simulink model "Linear_model"  (R2023a)
settings: Solver=VariableStepAuto  StartTime=0.0  StopTime=10.0  RelTol=1e-3
undefined symbols (not defined in the file): A, B, C, K
settings Model: Creator=jonat  LastModifiedBy=jonat

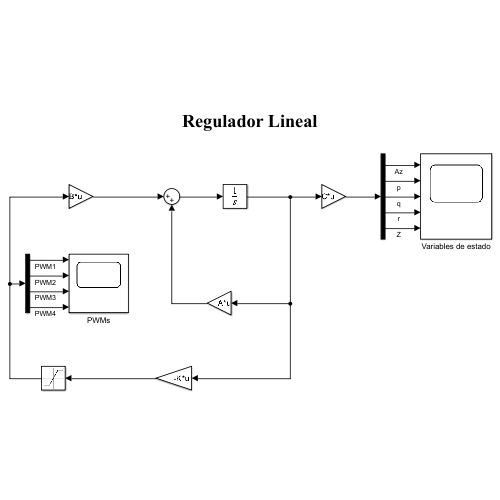
[thumbnail: Simulink's stored preview of the top-level diagram]
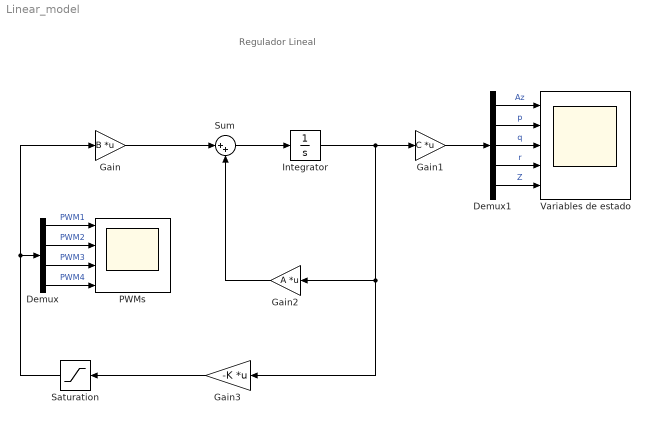
== system Linear_model ==
  note: Regulador Lineal
  Demux : Demux
  Demux1 : Demux  Outputs=5
  Gain : Gain  Gain=B  Multiplication=Matrix(K*u)
  Gain1 : Gain  Gain=C  Multiplication=Matrix(K*u)
  Gain2 : Gain  Gain=A  Multiplication=Matrix(K*u)
  Gain3 : Gain  Gain=-K  Multiplication=Matrix(K*u)
  Integrator : Integrator  InitialCondition=[0 0 0 0 1]
  PWMs : Scope  NumInputPorts=4
  Saturation : Saturate  UpperLimit=2e-3  LowerLimit=-2e-3
  Sum : Sum  Inputs=|++
  Variables de estado : Scope  NumInputPorts=5
  wires:
  Integrator/1 -> Gain3/1, Gain2/1, Gain1/1
  Gain/1 -> Sum/1
  Sum/1 -> Integrator/1
  Gain2/1 -> Sum/2
  Gain3/1 -> Saturation/1
  Saturation/1 -> Gain/1, Demux/1
  Demux/1 -> PWMs/1  "PWM1"
  Demux/2 -> PWMs/2  "PWM2"
  Demux/3 -> PWMs/3  "PWM3"
  Demux/4 -> PWMs/4  "PWM4"
  Demux1/1 -> Variables de estado/1  "Az"
  Demux1/2 -> Variables de estado/2  "p"
  Demux1/3 -> Variables de estado/3  "q"
  Demux1/4 -> Variables de estado/4  "r"
  Demux1/5 -> Variables de estado/5  "Z"
  Gain1/1 -> Demux1/1
